simulink model "TestNNMPC"  (R2020b)
settings: Solver=VariableStepAuto  StartTime=0.0  StopTime=10.0  RelTol=1e-3
undefined symbols (not defined in the file): A, B, C, D
libraries: neural x41, mpclib x1
(part 2 of 2)

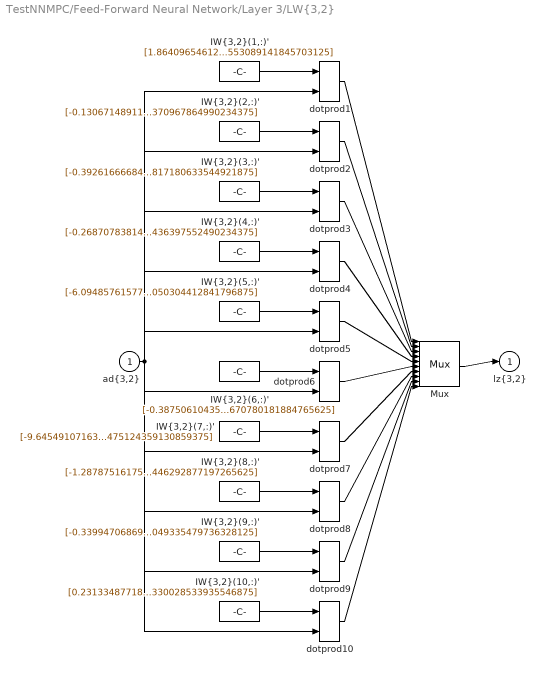
== system TestNNMPC/Feed-Forward Neural Network/Layer 3/LW{3,2} ==
  "ad{3,2}" : Inport  PortDimensions=10
      mask Display: e = 0.06;c1 = [120 230 180]/255;c2 = ([120 230 180]+0)/(256+128);c3 = ([120 230 180]+128)/(256+128);patch([0 1 1 0],[0 0 1 1],c1);patch([0 1 1 1-e 1-e 0+e],[0 0 1 1-e 0+e 0+e],c2);patch([0 0 1 1-e 0+e 0+e],[0 1 1 1-e 1-e 0+e],c3);plot([0 1 1 0 0],[0 0 1 1 0]);
  "IW{3,2}(1,:)'" : Constant  Value=[1.8640965461242302581013063900172710418701171875;-4.58811602434378063009035031427629292011260986328125;-5.99728214375561652360602238331921398639678955078125;-4.62332293016634476856552282697521150112152099609375;-3.06352919658799205393506781547330319881439208984375;6.09148721209460664027801612974144518375396728515625;10.0609334818987239401621991419233381748199462890625;-1.953972858970576265136287474888376891613006591796875;-12.806742744854176407898194156587123870849609375;-1.134561208504348162051655890536494553089141845703125]
      mask Display: e = 0.06;c1 = [120 150 230]/255;c2 = ([120 150 230]+0)/383;c3 = ([120 150 230]+128)/383;patch([0 1 1 0],[0 0 1 1],c1);patch([0 1 1 1-e 1-e 0+e],[0 0 1 1-e 0+e 0+e],c2);patch([0 0 1 1-e 0+e 0+e],[0 1 1 1-e 1-e 0+e],c3);plot([0 1 1 0 0],[0 0 1 1 0]);disp('weights');
  "IW{3,2}(10,:)'" : Constant  Value=[0.2313348771819067895005872514957445673644542694091796875;-0.237971529341388043921057260376983322203159332275390625;-1.5104740111113958977995253007975406944751739501953125;0.2422276702745886634016159177917870692908763885498046875;0.75460424019564964481787683325819671154022216796875;0.86117090087356285010855572181753814220428466796875;-2.07753399089241241881609312258660793304443359375;-0.2882799909649396141730903764255344867706298828125;0.5400867390923054234264100159634836018085479736328125;-0.50286964951270629597956940415315330028533935546875]
      mask Display: e = 0.06;c1 = [120 150 230]/255;c2 = ([120 150 230]+0)/383;c3 = ([120 150 230]+128)/383;patch([0 1 1 0],[0 0 1 1],c1);patch([0 1 1 1-e 1-e 0+e],[0 0 1 1-e 0+e 0+e],c2);patch([0 0 1 1-e 0+e 0+e],[0 1 1 1-e 1-e 0+e],c3);plot([0 1 1 0 0],[0 0 1 1 0]);disp('weights');
  "IW{3,2}(2,:)'" : Constant  Value=[-0.1306714891185073168511365793165168724954128265380859375;3.5384629655380219759308602078817784786224365234375;0.0292014895697302913346593555843355716206133365631103515625;0.486383931122554236115007597618387080729007720947265625;0.78807943351542686372113166726194322109222412109375;0.012957963289643416315843893471537739969789981842041015625;0.10924451130996522263405523744950187392532825469970703125;0.02833680267033444888369331238209269940853118896484375;0.7434646781468579046503464269335381686687469482421875;0.83265616416105225905397446695133112370967864990234375]
      mask Display: e = 0.06;c1 = [120 150 230]/255;c2 = ([120 150 230]+0)/383;c3 = ([120 150 230]+128)/383;patch([0 1 1 0],[0 0 1 1],c1);patch([0 1 1 1-e 1-e 0+e],[0 0 1 1-e 0+e 0+e],c2);patch([0 0 1 1-e 0+e 0+e],[0 1 1 1-e 1-e 0+e],c3);plot([0 1 1 0 0],[0 0 1 1 0]);disp('weights');
  "IW{3,2}(3,:)'" : Constant  Value=[-0.392616666845329920221274733194150030612945556640625;2.61200550215597093739461342920549213886260986328125;1.9448306539727193698041673997067846357822418212890625;0.53841607819010228741518631068174727261066436767578125;0.96713378076360101420760884138871915638446807861328125;-3.701370238837786263985663026687689125537872314453125;-3.505223667188229086377759813331067562103271484375;-0.58075909860817820362655083954450674355030059814453125;0.4078915728020462427849679443170316517353057861328125;-4.0771216250156907534574202145449817180633544921875]
      mask Display: e = 0.06;c1 = [120 150 230]/255;c2 = ([120 150 230]+0)/383;c3 = ([120 150 230]+128)/383;patch([0 1 1 0],[0 0 1 1],c1);patch([0 1 1 1-e 1-e 0+e],[0 0 1 1-e 0+e 0+e],c2);patch([0 0 1 1-e 0+e 0+e],[0 1 1 1-e 1-e 0+e],c3);plot([0 1 1 0 0],[0 0 1 1 0]);disp('weights');
  "IW{3,2}(4,:)'" : Constant  Value=[-0.2687078381466931897847416621516458690166473388671875;-1.93244667113590207208062565769068896770477294921875;2.35670994576424330801955875358544290065765380859375;0.271994646424023323039165234149550087749958038330078125;-0.23749092011509354005482919092173688113689422607421875;-0.61064253821969838309513534113648347556591033935546875;1.369957513156801365283854465815238654613494873046875;-0.94556223456629151513652686844579875469207763671875;-1.562334981659187160829560525598935782909393310546875;1.5316610468690450286288751158281229436397552490234375]
      mask Display: e = 0.06;c1 = [120 150 230]/255;c2 = ([120 150 230]+0)/383;c3 = ([120 150 230]+128)/383;patch([0 1 1 0],[0 0 1 1],c1);patch([0 1 1 1-e 1-e 0+e],[0 0 1 1-e 0+e 0+e],c2);patch([0 0 1 1-e 0+e 0+e],[0 1 1 1-e 1-e 0+e],c3);plot([0 1 1 0 0],[0 0 1 1 0]);disp('weights');
  "IW{3,2}(5,:)'" : Constant  Value=[-6.09485761577802964694683396373875439167022705078125;1.24606871499206750542043664609082043170928955078125;-2.784751607757535385445635256473906338214874267578125;3.231740517269958701263021794147789478302001953125;0.241982543833155594459327630829648114740848541259765625;2.4499290555645103495407965965569019317626953125;5.0122889803040688860846785246394574642181396484375;3.683767542261341620957182385609485208988189697265625;0.90466218662573416597894038204685784876346588134765625;2.78753626462389814122388997930102050304412841796875]
      mask Display: e = 0.06;c1 = [120 150 230]/255;c2 = ([120 150 230]+0)/383;c3 = ([120 150 230]+128)/383;patch([0 1 1 0],[0 0 1 1],c1);patch([0 1 1 1-e 1-e 0+e],[0 0 1 1-e 0+e 0+e],c2);patch([0 0 1 1-e 0+e 0+e],[0 1 1 1-e 1-e 0+e],c3);plot([0 1 1 0 0],[0 0 1 1 0]);disp('weights');
  "IW{3,2}(6,:)'" : Constant  Value=[-0.38750610435101717765604689702740870416164398193359375;-0.3687312832379967542095755561604164540767669677734375;0.0441945422003249266396096572862006723880767822265625;-0.07493036142117372178095280332854599691927433013916015625;0.381280499465895872379661568629671819508075714111328125;0.083941246119560386507174598591518588364124298095703125;0.5646495970748783843617957245442084968090057373046875;0.10543259965605054906401250036651617847383022308349609375;-1.4103920980615234359589749146834947168827056884765625;0.76142495589839731540138245691196061670780181884765625]
      mask Display: e = 0.06;c1 = [120 150 230]/255;c2 = ([120 150 230]+0)/383;c3 = ([120 150 230]+128)/383;patch([0 1 1 0],[0 0 1 1],c1);patch([0 1 1 1-e 1-e 0+e],[0 0 1 1-e 0+e 0+e],c2);patch([0 0 1 1-e 0+e 0+e],[0 1 1 1-e 1-e 0+e],c3);plot([0 1 1 0 0],[0 0 1 1 0]);disp('weights');
  "IW{3,2}(7,:)'" : Constant  Value=[-9.6454910716330086728476089774630963802337646484375;-16.430675384857298837459893547929823398590087890625;3.030841303894504346061467003892175853252410888671875;4.19054004083043540873632082366384565830230712890625;-3.397510914005290150186056052916683256626129150390625;0.58666391047018018323200294616981409490108489990234375;7.910216224829920150796169764362275600433349609375;3.892537408143202259935833353665657341480255126953125;-0.929386947564464716009524636319838464260101318359375;-4.35532505835590821874347966513596475124359130859375]
      mask Display: e = 0.06;c1 = [120 150 230]/255;c2 = ([120 150 230]+0)/383;c3 = ([120 150 230]+128)/383;patch([0 1 1 0],[0 0 1 1],c1);patch([0 1 1 1-e 1-e 0+e],[0 0 1 1-e 0+e 0+e],c2);patch([0 0 1 1-e 0+e 0+e],[0 1 1 1-e 1-e 0+e],c3);plot([0 1 1 0 0],[0 0 1 1 0]);disp('weights');
  "IW{3,2}(8,:)'" : Constant  Value=[-1.28787516175895522252403679885901510715484619140625;-1.94584821455145462465452510514296591281890869140625;0.1738031681709873155217138673833687789738178253173828125;0.321582125664233886563891928744851611554622650146484375;-0.350488609343190926637134907650761306285858154296875;0.86241577647043643484181529856869019567966461181640625;-0.2946373266035784421745802319492213428020477294921875;1.1875821220586946225239444174803793430328369140625;-0.0271585346357236280534497296912377350963652133941650390625;-0.2949007479320278068968264051363803446292877197265625]
      mask Display: e = 0.06;c1 = [120 150 230]/255;c2 = ([120 150 230]+0)/383;c3 = ([120 150 230]+128)/383;patch([0 1 1 0],[0 0 1 1],c1);patch([0 1 1 1-e 1-e 0+e],[0 0 1 1-e 0+e 0+e],c2);patch([0 0 1 1-e 0+e 0+e],[0 1 1 1-e 1-e 0+e],c3);plot([0 1 1 0 0],[0 0 1 1 0]);disp('weights');
  "IW{3,2}(9,:)'" : Constant  Value=[-0.339947068692762088826242461436777375638484954833984375;0.69767404026796120408704382498399354517459869384765625;-0.1295571597834702382012750376816256903111934661865234375;0.67302814384099385325299635951523669064044952392578125;0.1329938271153412732150655983787146396934986114501953125;0.140170661963239850944518138931016437709331512451171875;0.78873953722592970994043071186752058565616607666015625;0.2280464559773043020651783763241837732493877410888671875;-0.09712991007064201987031282214957172982394695281982421875;0.521952349401658910466039742459543049335479736328125]
      mask Display: e = 0.06;c1 = [120 150 230]/255;c2 = ([120 150 230]+0)/383;c3 = ([120 150 230]+128)/383;patch([0 1 1 0],[0 0 1 1],c1);patch([0 1 1 1-e 1-e 0+e],[0 0 1 1-e 0+e 0+e],c2);patch([0 0 1 1-e 0+e 0+e],[0 1 1 1-e 1-e 0+e],c3);plot([0 1 1 0 0],[0 0 1 1 0]);disp('weights');
  Mux : Mux  Inputs=10
      mask Display: e = 0.06;c1 = [120 150 230]/255;c2 = ([120 150 230]+0)/383;c3 = ([120 150 230]+128)/383;patch([0 1 1 0],[0 0 1 1],c1);patch([0 1 1 1-e 1-e 0+e],[0 0 1 1-e 0+e 0+e],c2);patch([0 0 1 1-e 0+e 0+e],[0 1 1 1-e 1-e 0+e],c3);plot([0 1 1 0 0],[0 0 1 1 0]);disp('Mux');
  dotprod{1..10} (10 alike) : neural/Weight Functions/dotprod
  "lz{3,2}" : Outport
      mask Display: e = 0.06;c1 = [120 230 180]/255;c2 = ([120 230 180]+0)/(256+128);c3 = ([120 230 180]+128)/(256+128);patch([0 1 1 0],[0 0 1 1],c1);patch([0 1 1 1-e 1-e 0+e],[0 0 1 1-e 0+e 0+e],c2);patch([0 0 1 1-e 0+e 0+e],[0 1 1 1-e 1-e 0+e],c3);plot([0 1 1 0 0],[0 0 1 1 0]);
  wires:
  "IW{3,2}(1,:)'"/1 -> dotprod1/1
  "ad{3,2}"/1 -> dotprod1/2, dotprod2/2, dotprod3/2, dotprod4/2, dotprod5/2, dotprod6/2, dotprod7/2, dotprod8/2, dotprod9/2, dotprod10/2
  dotprod1/1 -> Mux/1
  "IW{3,2}(2,:)'"/1 -> dotprod2/1
  dotprod2/1 -> Mux/2
  "IW{3,2}(3,:)'"/1 -> dotprod3/1
  dotprod3/1 -> Mux/3
  "IW{3,2}(4,:)'"/1 -> dotprod4/1
  dotprod4/1 -> Mux/4
  "IW{3,2}(5,:)'"/1 -> dotprod5/1
  dotprod5/1 -> Mux/5
  "IW{3,2}(6,:)'"/1 -> dotprod6/1
  dotprod6/1 -> Mux/6
  "IW{3,2}(7,:)'"/1 -> dotprod7/1
  dotprod7/1 -> Mux/7
  "IW{3,2}(8,:)'"/1 -> dotprod8/1
  dotprod8/1 -> Mux/8
  "IW{3,2}(9,:)'"/1 -> dotprod9/1
  dotprod9/1 -> Mux/9
  "IW{3,2}(10,:)'"/1 -> dotprod10/1
  dotprod10/1 -> Mux/10
  Mux/1 -> "lz{3,2}"/1

== system TestNNMPC/Feed-Forward Neural Network/Layer 4/Delays 1 ==
  "p{4}" : Inport  PortDimensions=10
      mask Display: e = 0.06;c1 = [120 230 180]/255;c2 = ([120 230 180]+0)/(256+128);c3 = ([120 230 180]+128)/(256+128);patch([0 1 1 0],[0 0 1 1],c1);patch([0 1 1 1-e 1-e 0+e],[0 0 1 1-e 0+e 0+e],c2);patch([0 0 1 1-e 0+e 0+e],[0 1 1 1-e 1-e 0+e],c3);plot([0 1 1 0 0],[0 0 1 1 0]);
  mux : Mux  Inputs=1
      mask Display: e = 0.06;c1 = [120 150 230]/255;c2 = ([120 150 230]+0)/383;c3 = ([120 150 230]+128)/383;patch([0 1 1 0],[0 0 1 1],c1);patch([0 1 1 1-e 1-e 0+e],[0 0 1 1-e 0+e 0+e],c2);patch([0 0 1 1-e 0+e 0+e],[0 1 1 1-e 1-e 0+e],c3);plot([0 1 1 0 0],[0 0 1 1 0]);disp('Mux')
  "pd{4,3}" : Outport
      mask Display: e = 0.06;c1 = [120 230 180]/255;c2 = ([120 230 180]+0)/(256+128);c3 = ([120 230 180]+128)/(256+128);patch([0 1 1 0],[0 0 1 1],c1);patch([0 1 1 1-e 1-e 0+e],[0 0 1 1-e 0+e 0+e],c2);patch([0 0 1 1-e 0+e 0+e],[0 1 1 1-e 1-e 0+e],c3);plot([0 1 1 0 0],[0 0 1 1 0]);
  wires:
  "p{4}"/1 -> mux/1
  mux/1 -> "pd{4,3}"/1

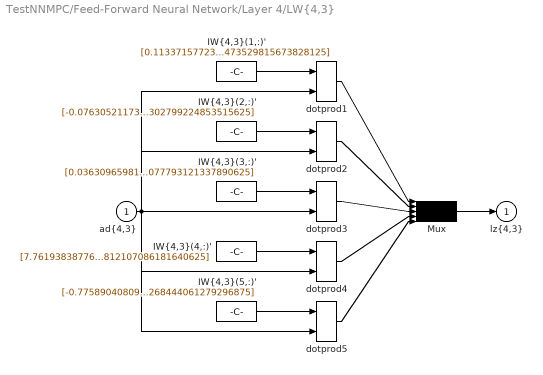
== system TestNNMPC/Feed-Forward Neural Network/Layer 4/LW{4,3} ==
  "ad{4,3}" : Inport  PortDimensions=10
      mask Display: e = 0.06;c1 = [120 230 180]/255;c2 = ([120 230 180]+0)/(256+128);c3 = ([120 230 180]+128)/(256+128);patch([0 1 1 0],[0 0 1 1],c1);patch([0 1 1 1-e 1-e 0+e],[0 0 1 1-e 0+e 0+e],c2);patch([0 0 1 1-e 0+e 0+e],[0 1 1 1-e 1-e 0+e],c3);plot([0 1 1 0 0],[0 0 1 1 0]);
  "IW{4,3}(1,:)'" : Constant  Value=[0.11337157723032635636695175662680412642657756805419921875;-2.505596887198360267490215846919454634189605712890625;-0.100929430516543294782394468711572699248790740966796875;0.0144740945939688982202486755568315857090055942535400390625;-0.04260946528416949263817770088280667550861835479736328125;1.3121730792163328604971184176974929869174957275390625;0.63463025510981918575481586231035180389881134033203125;0.4272870529471723965997398408944718539714813232421875;-0.98690767700485537705645811001886613667011260986328125;0.052622675851213884801182985029299743473529815673828125]
      mask Display: e = 0.06;c1 = [120 150 230]/255;c2 = ([120 150 230]+0)/383;c3 = ([120 150 230]+128)/383;patch([0 1 1 0],[0 0 1 1],c1);patch([0 1 1 1-e 1-e 0+e],[0 0 1 1-e 0+e 0+e],c2);patch([0 0 1 1-e 0+e 0+e],[0 1 1 1-e 1-e 0+e],c3);plot([0 1 1 0 0],[0 0 1 1 0]);disp('weights');
  "IW{4,3}(2,:)'" : Constant  Value=[-0.07630521173924161015822420495169353671371936798095703125;-2.259296408321230575921845229458995163440704345703125;-0.11191523420854716797112615722653572447597980499267578125;-0.1450091080208400218243269819140550680458545684814453125;0.00985184560082472647601914417236912413500249385833740234375;1.3590707364440579585362911529955454170703887939453125;0.53336062146574636511076050737756304442882537841796875;0.5383657221357449618182045014691539108753204345703125;-1.0042672853230436569305084049119614064693450927734375;-0.10359242938528469279990673612701357342302799224853515625]
      mask Display: e = 0.06;c1 = [120 150 230]/255;c2 = ([120 150 230]+0)/383;c3 = ([120 150 230]+128)/383;patch([0 1 1 0],[0 0 1 1],c1);patch([0 1 1 1-e 1-e 0+e],[0 0 1 1-e 0+e 0+e],c2);patch([0 0 1 1-e 0+e 0+e],[0 1 1 1-e 1-e 0+e],c3);plot([0 1 1 0 0],[0 0 1 1 0]);disp('weights');
  "IW{4,3}(3,:)'" : Constant  Value=[0.036309659818326546487643469163231202401220798492431640625;-2.29023467270874103718369951820932328701019287109375;-0.2060545034936335506703386499793850816786289215087890625;-0.045338850296719586385751910029284772463142871856689453125;-0.0189947337792961030988880821723796543665230274200439453125;1.24639665465734861271585032227449119091033935546875;-0.056027309360500439361363334000998293049633502960205078125;0.770927568194419432501263145240955054759979248046875;-1.0577570115042085330259169495548121631145477294921875;0.0237584004166173957950380923875854932703077793121337890625]
      mask Display: e = 0.06;c1 = [120 150 230]/255;c2 = ([120 150 230]+0)/383;c3 = ([120 150 230]+128)/383;patch([0 1 1 0],[0 0 1 1],c1);patch([0 1 1 1-e 1-e 0+e],[0 0 1 1-e 0+e 0+e],c2);patch([0 0 1 1-e 0+e 0+e],[0 1 1 1-e 1-e 0+e],c3);plot([0 1 1 0 0],[0 0 1 1 0]);disp('weights');
  "IW{4,3}(4,:)'" : Constant  Value=[7.7619383877656364053611304232305201367125846445560455322265625e-05;-2.9891321073577099554086089483462274074554443359375;-0.0939908006246479299505836024763993918895721435546875;-0.05711934726437851994607086680844076909124851226806640625;0.01387058688808262378600044684162639896385371685028076171875;1.474227970899914641478289922815747559070587158203125;0.96754844946673024264072182631934992969036102294921875;-0.141970258775600266520910963663482107222080230712890625;-0.80284174343378300608975450813886709511280059814453125;-0.072855159498319610467120810426422394812107086181640625]
      mask Display: e = 0.06;c1 = [120 150 230]/255;c2 = ([120 150 230]+0)/383;c3 = ([120 150 230]+128)/383;patch([0 1 1 0],[0 0 1 1],c1);patch([0 1 1 1-e 1-e 0+e],[0 0 1 1-e 0+e 0+e],c2);patch([0 0 1 1-e 0+e 0+e],[0 1 1 1-e 1-e 0+e],c3);plot([0 1 1 0 0],[0 0 1 1 0]);disp('weights');
  "IW{4,3}(5,:)'" : Constant  Value=[-0.77589040809248766006334108169539831578731536865234375;0.374960571450914381674834885416203178465366363525390625;-0.290557065232700473256244322328711859881877899169921875;-0.69560904563396330768654252096894197165966033935546875;0.0985724064547417733184175858696107752621173858642578125;-0.9121542733370866518072261897032149136066436767578125;-1.1981067546329455808518105186522006988525390625;1.1879814890141842109727576826117001473903656005859375;0.96650271685938360377576827886514365673065185546875;-0.68401862261994128555642191713559441268444061279296875]
      mask Display: e = 0.06;c1 = [120 150 230]/255;c2 = ([120 150 230]+0)/383;c3 = ([120 150 230]+128)/383;patch([0 1 1 0],[0 0 1 1],c1);patch([0 1 1 1-e 1-e 0+e],[0 0 1 1-e 0+e 0+e],c2);patch([0 0 1 1-e 0+e 0+e],[0 1 1 1-e 1-e 0+e],c3);plot([0 1 1 0 0],[0 0 1 1 0]);disp('weights');
  Mux : Mux  Inputs=5
      mask Display: e = 0.06;c1 = [120 150 230]/255;c2 = ([120 150 230]+0)/383;c3 = ([120 150 230]+128)/383;patch([0 1 1 0],[0 0 1 1],c1);patch([0 1 1 1-e 1-e 0+e],[0 0 1 1-e 0+e 0+e],c2);patch([0 0 1 1-e 0+e 0+e],[0 1 1 1-e 1-e 0+e],c3);plot([0 1 1 0 0],[0 0 1 1 0]);disp('Mux');
  dotprod{1..5} (5 alike) : neural/Weight Functions/dotprod
  "lz{4,3}" : Outport
      mask Display: e = 0.06;c1 = [120 230 180]/255;c2 = ([120 230 180]+0)/(256+128);c3 = ([120 230 180]+128)/(256+128);patch([0 1 1 0],[0 0 1 1],c1);patch([0 1 1 1-e 1-e 0+e],[0 0 1 1-e 0+e 0+e],c2);patch([0 0 1 1-e 0+e 0+e],[0 1 1 1-e 1-e 0+e],c3);plot([0 1 1 0 0],[0 0 1 1 0]);
  wires:
  "IW{4,3}(1,:)'"/1 -> dotprod1/1
  "ad{4,3}"/1 -> dotprod1/2, dotprod2/2, dotprod3/2, dotprod4/2, dotprod5/2
  dotprod1/1 -> Mux/1
  "IW{4,3}(2,:)'"/1 -> dotprod2/1
  dotprod2/1 -> Mux/2
  "IW{4,3}(3,:)'"/1 -> dotprod3/1
  dotprod3/1 -> Mux/3
  "IW{4,3}(4,:)'"/1 -> dotprod4/1
  dotprod4/1 -> Mux/4
  "IW{4,3}(5,:)'"/1 -> dotprod5/1
  dotprod5/1 -> Mux/5
  Mux/1 -> "lz{4,3}"/1
